simulink model "pH2Oslx"  (R2023a)
settings: Solver=VariableStepAuto  StartTime=0.0  StopTime=10.0  RelTol=1e-3
settings Model: Creator=meghn  LastModifiedBy=meghn

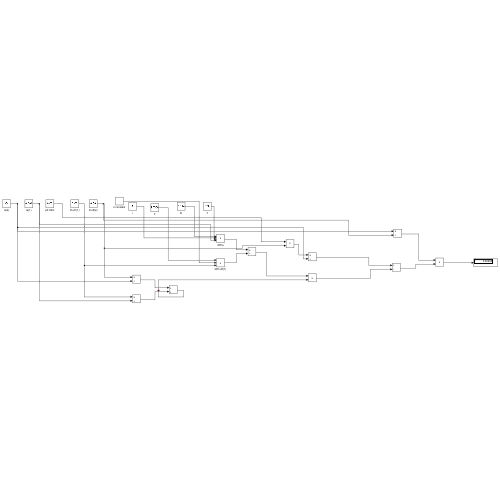
[thumbnail: Simulink's stored preview of the top-level diagram]
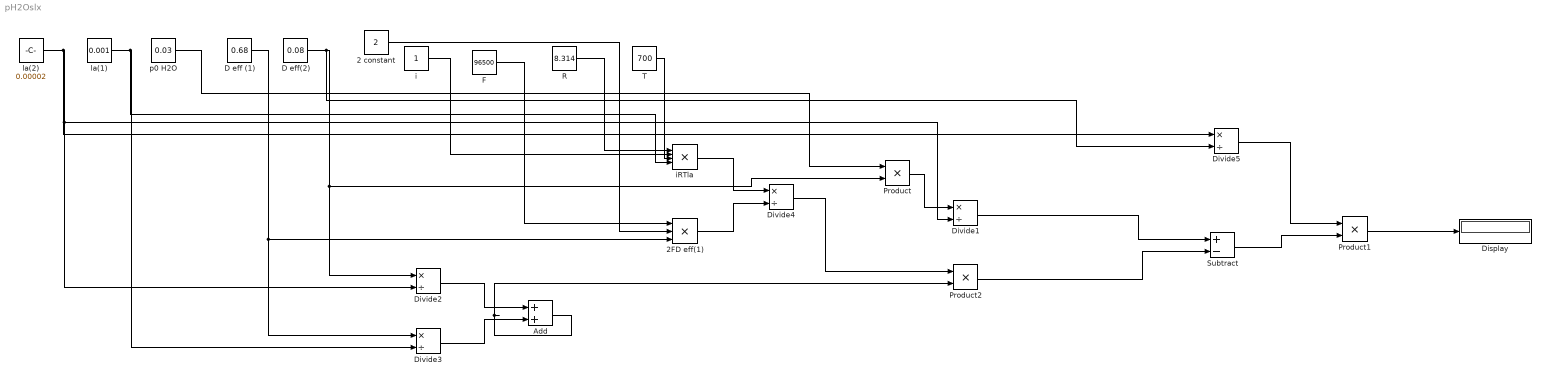
== system pH2Oslx ==
  2 constant : Constant  Value=2
  2FD eff(1) : Product  Inputs=3  RndMeth=Round
  Add : Sum
  D eff (1) : Constant  Value=0.68
  D eff(2) : Constant  Value=0.08
  Display : Display
  Divide{1..5} (5 alike) : Product  Inputs=*/
  F : Constant  Value=96500
  Product : Product
  Product1 : Product
  Product2 : Product
  R : Constant  Value=8.314
  Subtract : Sum  Inputs=+-
  T : Constant  Value=700
  i : Constant
  iRTla : Product  Inputs=4
  la(1) : Constant  Value=0.001
  la(2) : Constant  Value=0.00002
  p0 H2O : Constant  Value=0.03
  wires:
  Divide4/1 -> Product2/1
  Product1/1 -> Display/1
  2FD eff(1)/1 -> Divide4/2
  Divide3/1 -> Add/2
  la(1)/1 -> iRTla/4, Divide3/2
  R/1 -> iRTla/1
  Divide2/1 -> Add/1
  Add/1 -> Product2/2
  Product2/1 -> Subtract/2
  T/1 -> iRTla/3
  la(2)/1 -> Divide5/1, Divide2/2, Divide1/2
  Divide5/1 -> Product1/1
  Subtract/1 -> Product1/2
  p0 H2O/1 -> Product/1
  iRTla/1 -> Divide4/1
  D eff(2)/1 -> Divide5/2, Divide2/1, Product/2
  F/1 -> 2FD eff(1)/1
  D eff (1)/1 -> 2FD eff(1)/3, Divide3/1
  Divide1/1 -> Subtract/1
  Product/1 -> Divide1/1
  i/1 -> iRTla/2
  2 constant/1 -> 2FD eff(1)/2
